simulink model "Task_No6_Thermal"  (R2023b)
settings: Solver=ode5  StartTime=0.0  StopTime=3600*24*7  FixedStep=1  RelTol=1e-3
InitFcn:
  | PARAMETERS;
StartFcn:
  | PARAMETERS;
values from neighbouring files (symbols this model uses):
  Conv_C_to_K = 273.15    [PARAMETERS.m]
  P_AC_AIR_FLOW = 1    [PARAMETERS.m]
  P_AREA_BATH = 2*4    (= 8)    [PARAMETERS.m]
  P_AREA_BDR1 = 3.87^2    (= 14.9769)    [PARAMETERS.m]
  P_AREA_BDR2 = 3.87*4.5    (= 17.415)    [PARAMETERS.m]
  P_AREA_EAST_WALL_BATH = 2*P_RM_HEIGHT - P_AREA_WIN_BATH    (= 3.7)    [PARAMETERS.m]
  P_AREA_EAST_WALL_BDR2 = 3.87*P_RM_HEIGHT - P_AREA_WIN_BDRS    (= 7.075)    [PARAMETERS.m]
  P_AREA_EAST_WALL_KIT = 4.13*P_RM_HEIGHT    (= 10.325)    [PARAMETERS.m]
  P_AREA_HALL = 2*6    (= 12)    [PARAMETERS.m]
  P_AREA_KIT = 4.13*4    (= 16.52)    [PARAMETERS.m]
  P_AREA_LVR = 4.13*6    (= 24.78)    [PARAMETERS.m]
  P_AREA_NORTH_WALL_BATH = 1.63*P_RM_HEIGHT    (= 4.075)    [PARAMETERS.m]
  P_AREA_NORTH_WALL_BDR1 = 3.87*P_RM_HEIGHT - P_AREA_WIN_BDRS    (= 7.075)    [PARAMETERS.m]
  P_AREA_NORTH_WALL_BDR2 = 4.5*P_RM_HEIGHT - P_AREA_WIN_BDRS    (= 8.65)    [PARAMETERS.m]
  P_AREA_OUTER_WALL_BATH = (1.63+2)*P_RM_HEIGHT - P_AREA_WIN_BATH    (= 7.775)    [PARAMETERS.m]
  P_AREA_OUTER_WALL_BDR1 = 3.87*2*P_RM_HEIGHT - P_AREA_WIN_BDRS    (= 16.75)    [PARAMETERS.m]
  P_AREA_OUTER_WALL_BDR2 = (4.5+3.87)*P_RM_HEIGHT - P_AREA_WIN_BDRS*2    (= 15.725)    [PARAMETERS.m]
  P_AREA_OUTER_WALL_HALL = 2*P_RM_HEIGHT - P_AREA_SING_DOOR    (= 2.9)    [PARAMETERS.m]
  P_AREA_OUTER_WALL_KIT = (4+4.13)*P_RM_HEIGHT - P_AREA_WIN_KIT    (= 13.725)    [PARAMETERS.m]
  P_AREA_OUTER_WALL_LVR = (4.13+6)*P_RM_HEIGHT - P_AREA_WIN_LVR    (= 14.325)    [PARAMETERS.m]
  P_AREA_SOUTH_WALL_KIT = 4*P_RM_HEIGHT - P_AREA_WIN_KIT    (= 3.4)    [PARAMETERS.m]
  P_AREA_SOUTH_WALL_LVR = 6*P_RM_HEIGHT - P_AREA_WIN_LVR    (= 4)    [PARAMETERS.m]
  P_AREA_WALL_BATH_KIT = 4*P_RM_HEIGHT    (= 10)    [PARAMETERS.m]
  P_AREA_WALL_BDR1_BDR2 = 3.87*P_RM_HEIGHT    (= 9.675)    [PARAMETERS.m]
  P_AREA_WALL_BDR1_HALL = 3.87*P_RM_HEIGHT - P_AREA_SING_DOOR    (= 7.575)    [PARAMETERS.m]
  P_AREA_WALL_BDR2_BATH = 2.37*P_RM_HEIGHT    (= 5.925)    [PARAMETERS.m]
  P_AREA_WALL_BDR2_HALL = 2.13*P_RM_HEIGHT - P_AREA_SING_DOOR    (= 3.225)    [PARAMETERS.m]
  P_AREA_WALL_HALL_BATH = 2*P_RM_HEIGHT - P_AREA_SING_DOOR    (= 2.9)    [PARAMETERS.m]
  P_AREA_WALL_HALL_LVR = 6*P_RM_HEIGHT - P_AREA_DBL_DOOR    (= 10.8)    [PARAMETERS.m]
  P_AREA_WALL_LVR_KIT = 4.13*P_RM_HEIGHT - P_AREA_DBL_DOOR    (= 6.125)    [PARAMETERS.m]
  P_AREA_WIN_BATH = P_H_WIN_NORM*P_W_WIN_BATH    (= 1.3)    [PARAMETERS.m]
  P_AREA_WIN_BDRS = P_H_WIN_NORM*P_W_WIN_BDRS    (= 2.6)    [PARAMETERS.m]
  P_AREA_WIN_KIT = P_H_WIN_DOOR*P_W_WIN_KIT    (= 6.6)    [PARAMETERS.m]
  P_AREA_WIN_LVR = P_H_WIN_DOOR*P_W_WIN_LVR    (= 11)    [PARAMETERS.m]
  P_CP_AIR = 1012    [PARAMETERS.m]
  P_DENSITY_BRICK = 2/(10^-3)    (= 2000)    [PARAMETERS.m]
  P_DENSITY_PUR = 150    [PARAMETERS.m]
  P_EM_GLASS = 0.94    [PARAMETERS.m]
  P_EM_WALL = 0.94    [PARAMETERS.m]
  P_HUMAN = 60    [PARAMETERS.m]
  P_M_WINDOW_SPEC = 20    [PARAMETERS.m]
  P_THICK_BRICK = 0.175    [PARAMETERS.m]
  P_THICK_PUR = P_THICK_WALL - P_THICK_BRICK    (= 0.125)    [PARAMETERS.m]
  T_COOLER = 12    [PARAMETERS.m]
  T_HEATER = 50    [PARAMETERS.m]
  T_INIT_BDR = 22    [PARAMETERS.m]
  T_INIT_OUT = 2.9    [PARAMETERS.m]
  U_CEIL = 1.1    [PARAMETERS.m]
  U_INNER_WALL_BR = 3    [PARAMETERS.m]
  U_INNER_WALL_PC = 0.6    [PARAMETERS.m]
  U_WALL = 0.32    [PARAMETERS.m]
  U_WINDOW = 3.0    (= 3)    [PARAMETERS.m]
undefined symbols (not defined in the file or in its folder): TBL_SOL_EAST_01, TBL_SOL_EAST_02, TBL_SOL_EAST_03, TBL_SOL_EAST_04, TBL_SOL_EAST_05, TBL_SOL_EAST_06, TBL_SOL_EAST_07, TBL_SOL_EAST_08, TBL_SOL_EAST_09, TBL_SOL_EAST_10, TBL_SOL_EAST_11, TBL_SOL_EAST_12, TBL_SOL_NORTH_01, TBL_SOL_NORTH_02, TBL_SOL_NORTH_03, TBL_SOL_NORTH_04, TBL_SOL_NORTH_05, TBL_SOL_NORTH_06, TBL_SOL_NORTH_07, TBL_SOL_NORTH_08, TBL_SOL_NORTH_09, TBL_SOL_NORTH_10, TBL_SOL_NORTH_11, TBL_SOL_NORTH_12, TBL_SOL_SOUTH_01, TBL_TEMP
libraries: fl_lib x135, nesl_utility x39, slpidlib x3
(part 2 of 3)

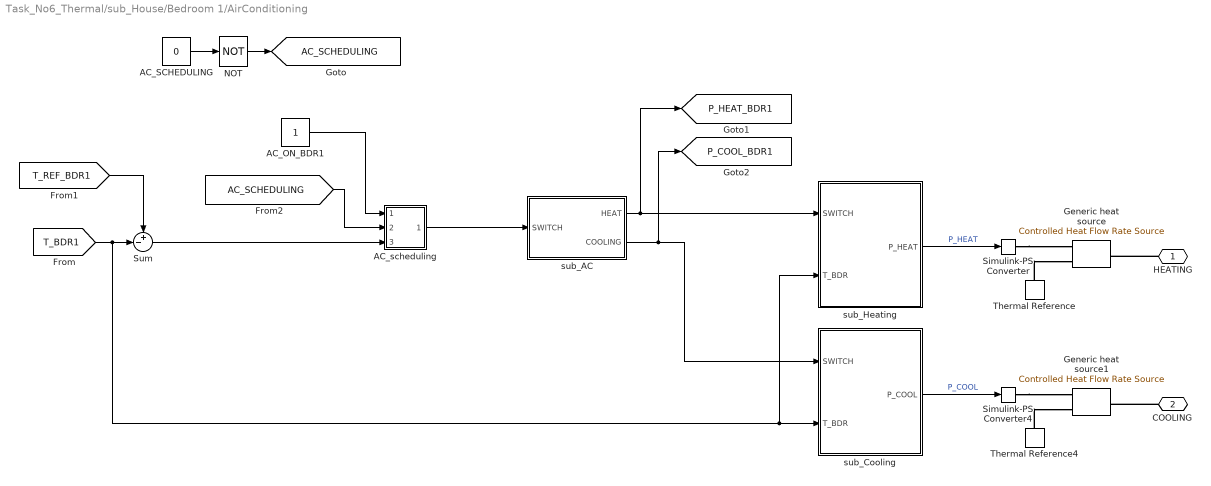
== system Task_No6_Thermal/sub_House/Bedroom 1/AirConditioning ==
  AC_ON_BDR1 : Constant
  AC_SCHEDULING : Constant  Value=0
  AC_scheduling : Subsystem
  Generic heat source : fl_lib/Thermal/Thermal Sources/Controlled Heat Flow Rate Source
  Generic heat source1 : fl_lib/Thermal/Thermal Sources/Controlled Heat Flow Rate Source
  NOT : Logic  Operator=NOT  IconShape=distinctive  AllPortsSameDT=off  OutDataTypeStr=boolean
  Simulink-PS Converter : nesl_utility/Simulink-PS Converter  PhysicalDomain=network_engine_domain  SubClassName=ps_input  LeftPortType=input  RightPortType=output  PseudoPeriodic=off  Frequencies=[]  NoiseDistribution=none  NoiseParameters=[]  Unit=1  AffineConversion=off  FilteringAndDerivatives=provide  SimscapeFilterOrder=1  InputFilterTimeConstant=0.001  UdotUserProvided=0
  Simulink-PS Converter4 : nesl_utility/Simulink-PS Converter  PhysicalDomain=network_engine_domain  SubClassName=ps_input  LeftPortType=input  RightPortType=output  PseudoPeriodic=off  Frequencies=[]  NoiseDistribution=none  NoiseParameters=[]  Unit=1  AffineConversion=off  FilteringAndDerivatives=provide  SimscapeFilterOrder=1  InputFilterTimeConstant=0.001  UdotUserProvided=0
  Sum : Sum  Inputs=+-|
  Thermal Reference : fl_lib/Thermal/Thermal Elements/Thermal Reference
  Thermal Reference4 : fl_lib/Thermal/Thermal Elements/Thermal Reference
  sub_AC : Subsystem
  sub_Cooling : Subsystem
  sub_Heating : Subsystem
  HEATING : PMIOPort  Side=Right
  COOLING : PMIOPort  Port=2  Side=Right
  tag scope: AC_SCHEDULING=global, P_COOL_BDR1=global, P_HEAT_BDR1=global
  wires:
  sub_AC/2(COOLING) -> [P_COOL_BDR1], sub_Cooling/1(SWITCH)
  sub_AC/1(HEAT) -> [P_HEAT_BDR1], sub_Heating/1(SWITCH)
  [T_BDR1] -> sub_Heating/2(T_BDR), sub_Cooling/2(T_BDR), Sum/2
  sub_Heating/1(P_HEAT) -> Simulink-PS Converter/1  "P_HEAT"
  sub_Cooling/1(P_COOL) -> Simulink-PS Converter4/1  "P_COOL"
  [T_REF_BDR1] -> Sum/1
  AC_ON_BDR1/1 -> AC_scheduling/1(In1)
  Sum/1 -> AC_scheduling/3(In2)
  AC_scheduling/1(Out1) -> sub_AC/1(SWITCH)
  AC_SCHEDULING/1 -> NOT/1
  [AC_SCHEDULING] -> AC_scheduling/2(In3)
  NOT/1 -> [AC_SCHEDULING]
  connections:
  Thermal Reference4/LConn1 -- Generic heat source1/RConn2
  Thermal Reference/LConn1 -- Generic heat source/RConn2
  Simulink-PS Converter4/RConn1 -- Generic heat source1/RConn1
  Simulink-PS Converter/RConn1 -- Generic heat source/RConn1
  HEATING/RConn1 -- Generic heat source/LConn1
  COOLING/RConn1 -- Generic heat source1/LConn1

== system Task_No6_Thermal/sub_House/Bedroom 1/Ceiling & Floor (BDR1<->Above & Below) ==
  Ceiling-InAir : fl_lib/Thermal/Thermal Elements/Thermal Resistance  resistance=1/(U_CEIL*P_AREA_BDR1) K/W  T_specify=off  T_priority=None  T=0 K  T_nominal_specify=off  T_nominal_unit=K  T_nominal_value=1  Q_specify=off  Q_priority=None  Q=0 W  Q_nominal_specify=off  Q_nominal_unit=W  Q_nominal_value=1
  Floor-InAir : fl_lib/Thermal/Thermal Elements/Thermal Resistance  resistance=1/(U_CEIL*P_AREA_BDR1) K/W  T_specify=off  T_priority=None  T=0 K  T_nominal_specify=off  T_nominal_unit=K  T_nominal_value=1  Q_specify=off  Q_priority=None  Q=0 W  Q_nominal_specify=off  Q_nominal_unit=W  Q_nominal_value=1
  Conn1 : PMIOPort  Side=Left
  Conn2 : PMIOPort  Port=2  Side=Right
  connections:
  Ceiling-InAir/RConn1 -- Conn2/RConn1 -- Floor-InAir/RConn1
  Ceiling-InAir/LConn1 -- Conn1/RConn1 -- Floor-InAir/LConn1

== system Task_No6_Thermal/sub_House/Bedroom 1/Heat source human ==
  Constant : Constant  Value=P_HUMAN
  Controlled Heat Flow Rate Source : fl_lib/Thermal/Thermal Sources/Controlled Heat Flow Rate Source
  Product : Product
  Simulink-PS Converter : nesl_utility/Simulink-PS Converter  PhysicalDomain=network_engine_domain  SubClassName=ps_input  LeftPortType=input  RightPortType=output  PseudoPeriodic=off  Frequencies=[]  NoiseDistribution=none  NoiseParameters=[]  Unit=1  AffineConversion=off  FilteringAndDerivatives=provide  SimscapeFilterOrder=1  InputFilterTimeConstant=0.001  UdotUserProvided=0
  Thermal Reference : fl_lib/Thermal/Thermal Elements/Thermal Reference
  Conn1 : PMIOPort  Side=Left
  wires:
  [N_BDR1] -> Product/1
  Constant/1 -> Product/2
  Product/1 -> Simulink-PS Converter/1
  connections:
  Thermal Reference/LConn1 -- Controlled Heat Flow Rate Source/RConn2
  Simulink-PS Converter/RConn1 -- Controlled Heat Flow Rate Source/RConn1
  Controlled Heat Flow Rate Source/LConn1 -- Conn1/RConn1

== system Task_No6_Thermal/sub_House/Bedroom 1/Inside Enivornment Temperature ==
  T_ENV : Inport
  Constant2 : Constant  Value=Conv_C_to_K
  Controlled Temperature Source : fl_lib/Thermal/Thermal Sources/Controlled Temperature Source
  Simulink-PS Converter1 : nesl_utility/Simulink-PS Converter  PhysicalDomain=network_engine_domain  SubClassName=ps_input  LeftPortType=input  RightPortType=output  PseudoPeriodic=off  Frequencies=[]  NoiseDistribution=none  NoiseParameters=[]  Unit=1  AffineConversion=off  FilteringAndDerivatives=provide  SimscapeFilterOrder=1  InputFilterTimeConstant=0.001  UdotUserProvided=0
  Sum : Sum  Inputs=|++
  Thermal Reference1 : fl_lib/Thermal/Thermal Elements/Thermal Reference
  Conn1 : PMIOPort  Side=Left
  wires:
  T_ENV/1 -> Sum/1
  Constant2/1 -> Sum/2
  Sum/1 -> Simulink-PS Converter1/1
  connections:
  Controlled Temperature Source/LConn1 -- Conn1/RConn1
  Simulink-PS Converter1/RConn1 -- Controlled Temperature Source/RConn1
  Thermal Reference1/LConn1 -- Controlled Temperature Source/RConn2

== system Task_No6_Thermal/sub_House/Bedroom 1/Outside Temperature ==
  T_OUT : Inport
  Constant2 : Constant  Value=Conv_C_to_K
  Controlled Temperature Source : fl_lib/Thermal/Thermal Sources/Controlled Temperature Source
  Simulink-PS Converter1 : nesl_utility/Simulink-PS Converter  PhysicalDomain=network_engine_domain  SubClassName=ps_input  LeftPortType=input  RightPortType=output  PseudoPeriodic=off  Frequencies=[]  NoiseDistribution=none  NoiseParameters=[]  Unit=1  AffineConversion=off  FilteringAndDerivatives=provide  SimscapeFilterOrder=1  InputFilterTimeConstant=0.001  UdotUserProvided=0
  Sum : Sum  Inputs=|++
  Thermal Reference1 : fl_lib/Thermal/Thermal Elements/Thermal Reference
  Conn1 : PMIOPort  Side=Left
  wires:
  Sum/1 -> Simulink-PS Converter1/1
  Constant2/1 -> Sum/2
  T_OUT/1 -> Sum/1
  connections:
  Thermal Reference1/LConn1 -- Controlled Temperature Source/RConn2
  Simulink-PS Converter1/RConn1 -- Controlled Temperature Source/RConn1
  Controlled Temperature Source/LConn1 -- Conn1/RConn1

== system Task_No6_Thermal/sub_House/Bedroom 1/SOLAR__WALL ==
  Constant : Constant  Value=P_AREA_NORTH_WALL_BDR1
  Constant1 : Constant  Value=P_EM_WALL
  Controlled Heat Flow Rate Source : fl_lib/Thermal/Thermal Sources/Controlled Heat Flow Rate Source
  Product : Product  Inputs=3
  Simulink-PS Converter : nesl_utility/Simulink-PS Converter  PhysicalDomain=network_engine_domain  SubClassName=ps_input  LeftPortType=input  RightPortType=output  PseudoPeriodic=off  Frequencies=[]  NoiseDistribution=none  NoiseParameters=[]  Unit=1  AffineConversion=off  FilteringAndDerivatives=provide  SimscapeFilterOrder=1  InputFilterTimeConstant=0.001  UdotUserProvided=0
  Thermal Reference : fl_lib/Thermal/Thermal Elements/Thermal Reference
  Conn1 : PMIOPort  Side=Left
  wires:
  Constant/1 -> Product/2
  Constant1/1 -> Product/1
  [SOL_NORTH] -> Product/3
  Product/1 -> Simulink-PS Converter/1
  connections:
  Controlled Heat Flow Rate Source/LConn1 -- Conn1/RConn1
  Simulink-PS Converter/RConn1 -- Controlled Heat Flow Rate Source/RConn1
  Thermal Reference/LConn1 -- Controlled Heat Flow Rate Source/RConn2

== system Task_No6_Thermal/sub_House/Bedroom 1/SOLAR__WINDOW ==
  Constant : Constant  Value=P_AREA_WIN_BDRS
  Constant1 : Constant  Value=P_EM_GLASS
  Controlled Heat Flow Rate Source : fl_lib/Thermal/Thermal Sources/Controlled Heat Flow Rate Source
  Product : Product  Inputs=3
  Simulink-PS Converter : nesl_utility/Simulink-PS Converter  PhysicalDomain=network_engine_domain  SubClassName=ps_input  LeftPortType=input  RightPortType=output  PseudoPeriodic=off  Frequencies=[]  NoiseDistribution=none  NoiseParameters=[]  Unit=1  AffineConversion=off  FilteringAndDerivatives=provide  SimscapeFilterOrder=1  InputFilterTimeConstant=0.001  UdotUserProvided=0
  Thermal Reference : fl_lib/Thermal/Thermal Elements/Thermal Reference
  Conn1 : PMIOPort  Side=Left
  wires:
  Product/1 -> Simulink-PS Converter/1
  [SOL_NORTH] -> Product/3
  Constant1/1 -> Product/1
  Constant/1 -> Product/2
  connections:
  Thermal Reference/LConn1 -- Controlled Heat Flow Rate Source/RConn2
  Simulink-PS Converter/RConn1 -- Controlled Heat Flow Rate Source/RConn1
  Controlled Heat Flow Rate Source/LConn1 -- Conn1/RConn1

== system Task_No6_Thermal/sub_House/Bedroom 1/TEMP_01 ==
  Constant2 : Constant  Value=Conv_C_to_K
  PS-Simulink Converter : nesl_utility/PS-Simulink Converter  PhysicalDomain=network_engine_domain  SubClassName=ps_output  LeftPortType=input  RightPortType=output  PseudoPeriodic=off  Frequencies=[]  VectorFormat=inherit  Unit=inherit  AffineConversion=off
  Sum : Sum  Inputs=|+-
  Temperature Sensor : fl_lib/Thermal/Thermal Sensors/Temperature Sensor  temperature_measure=foundation.enum.MeasurementReference.difference
  Thermal Reference2 : fl_lib/Thermal/Thermal Elements/Thermal Reference
  PS : PMIOPort  Side=Left
  Sim : Outport
  wires:
  Sum/1 -> Sim/1
  PS-Simulink Converter/1 -> Sum/1
  Constant2/1 -> Sum/2
  connections:
  Thermal Reference2/LConn1 -- Temperature Sensor/RConn1
  PS-Simulink Converter/LConn1 -- Temperature Sensor/RConn2
  PS/RConn1 -- Temperature Sensor/LConn1

== system Task_No6_Thermal/sub_House/Bedroom 1/Wall (BDR1<->Outside) ==
  InAir-Wall : fl_lib/Thermal/Thermal Elements/Thermal Resistance  resistance=1/(U_WALL*P_AREA_OUTER_WALL_BDR1)/2 K/W  T_specify=off  T_priority=None  T=0 K  T_nominal_specify=off  T_nominal_unit=K  T_nominal_value=1  Q_specify=off  Q_priority=None  Q=0 W  Q_nominal_specify=off  Q_nominal_unit=W  Q_nominal_value=1
  Thermal Mass of wall : fl_lib/Thermal/Thermal Elements/Thermal Mass  mass_type=foundation.enum.constant_variable.constant  mass=P_AREA_OUTER_WALL_BDR1*(P_THICK_BRICK*P_DENSITY_BRICK+P_THICK_PUR*P_DENSITY_PUR) kg  sp_heat=P_CP_WALL J/(K*kg)  mass_min=1e-6 kg  num_ports=foundation.enum.numPorts2.one  m_specify=off  m_priority=High  m=1 kg  m_nominal_specify=off  m_nominal_unit=kg  m_nominal_value=1  T_specify=on  T_priority=High  T=T_INIT_BDR degC  T_nominal_specify=off  T_nominal_unit=K  T_nominal_value=1  Q_specify=off  Q_priority=None  Q=0 W  Q_nominal_specify=off  Q_nominal_unit=W  Q_nominal_value=1
  Wall-OutAir : fl_lib/Thermal/Thermal Elements/Thermal Resistance  resistance=1/(U_WALL*P_AREA_OUTER_WALL_BDR1)/2 K/W  T_specify=off  T_priority=None  T=0 K  T_nominal_specify=off  T_nominal_unit=K  T_nominal_value=1  Q_specify=off  Q_priority=None  Q=0 W  Q_nominal_specify=off  Q_nominal_unit=W  Q_nominal_value=1
  Conn1 : PMIOPort  Side=Left
  Conn3 : PMIOPort  Port=2  Side=Right
  Conn2 : PMIOPort  Port=3  Side=Right
  connections:
  Conn1/RConn1 -- InAir-Wall/LConn1
  InAir-Wall/RConn1 -- Conn3/RConn1 -- Thermal Mass of wall/LConn1 -- Wall-OutAir/LConn1
  Wall-OutAir/RConn1 -- Conn2/RConn1

== system Task_No6_Thermal/sub_House/Bedroom 1/Window (BDR1<->Outside) ==
  InAir-Window : fl_lib/Thermal/Thermal Elements/Thermal Resistance  resistance=1/(U_WINDOW*P_AREA_WIN_BDRS)/2 K/W  T_specify=off  T_priority=None  T=0 K  T_nominal_specify=off  T_nominal_unit=K  T_nominal_value=1  Q_specify=off  Q_priority=None  Q=0 W  Q_nominal_specify=off  Q_nominal_unit=W  Q_nominal_value=1
  Thermal Mass of window : fl_lib/Thermal/Thermal Elements/Thermal Mass  mass_type=foundation.enum.constant_variable.constant  mass=P_M_WINDOW_SPEC*P_AREA_WIN_BDRS kg  sp_heat=P_CP_GLASS J/(K*kg)  mass_min=1e-6 kg  num_ports=foundation.enum.numPorts2.one  m_specify=off  m_priority=High  m=1 kg  m_nominal_specify=off  m_nominal_unit=kg  m_nominal_value=1  T_specify=on  T_priority=High  T=T_INIT_BDR degC  T_nominal_specify=off  T_nominal_unit=K  T_nominal_value=1  Q_specify=off  Q_priority=None  Q=0 W  Q_nominal_specify=off  Q_nominal_unit=W  Q_nominal_value=1
  Window-OutAir : fl_lib/Thermal/Thermal Elements/Thermal Resistance  resistance=1/(U_WINDOW*P_AREA_WIN_BDRS)/2 K/W  T_specify=off  T_priority=None  T=0 K  T_nominal_specify=off  T_nominal_unit=K  T_nominal_value=1  Q_specify=off  Q_priority=None  Q=0 W  Q_nominal_specify=off  Q_nominal_unit=W  Q_nominal_value=1
  Conn1 : PMIOPort  Side=Right
  Conn2 : PMIOPort  Port=2  Side=Left
  Conn3 : PMIOPort  Port=3  Side=Right
  connections:
  Window-OutAir/LConn1 -- Thermal Mass of window/LConn1 -- Conn3/RConn1 -- InAir-Window/RConn1
  Conn1/RConn1 -- Window-OutAir/RConn1
  Conn2/RConn1 -- InAir-Window/LConn1

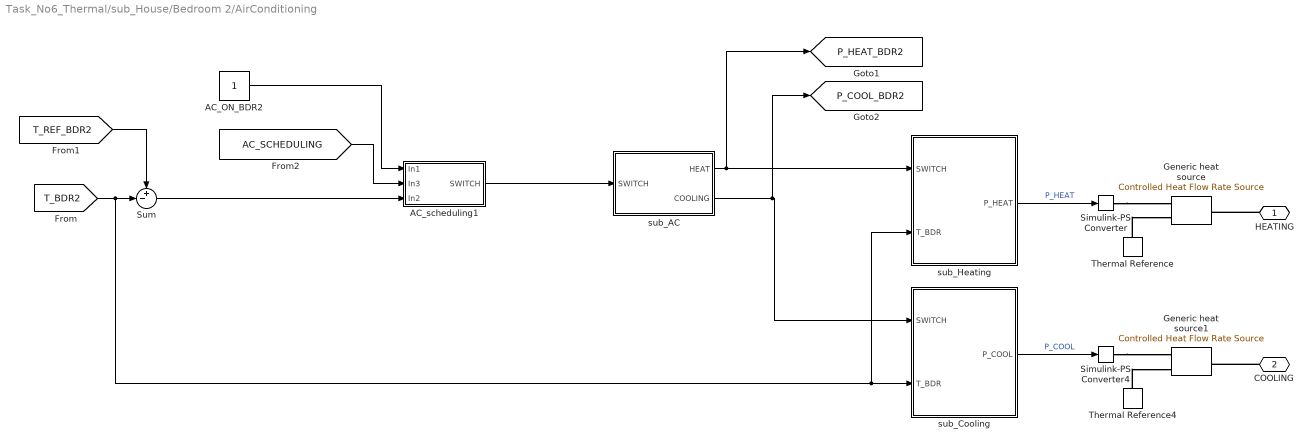
== system Task_No6_Thermal/sub_House/Bedroom 2/AirConditioning ==
  AC_ON_BDR2 : Constant
  AC_scheduling1 : Subsystem
  Generic heat source : fl_lib/Thermal/Thermal Sources/Controlled Heat Flow Rate Source
  Generic heat source1 : fl_lib/Thermal/Thermal Sources/Controlled Heat Flow Rate Source
  Simulink-PS Converter : nesl_utility/Simulink-PS Converter  PhysicalDomain=network_engine_domain  SubClassName=ps_input  LeftPortType=input  RightPortType=output  PseudoPeriodic=off  Frequencies=[]  NoiseDistribution=none  NoiseParameters=[]  Unit=1  AffineConversion=off  FilteringAndDerivatives=provide  SimscapeFilterOrder=1  InputFilterTimeConstant=0.001  UdotUserProvided=0
  Simulink-PS Converter4 : nesl_utility/Simulink-PS Converter  PhysicalDomain=network_engine_domain  SubClassName=ps_input  LeftPortType=input  RightPortType=output  PseudoPeriodic=off  Frequencies=[]  NoiseDistribution=none  NoiseParameters=[]  Unit=1  AffineConversion=off  FilteringAndDerivatives=provide  SimscapeFilterOrder=1  InputFilterTimeConstant=0.001  UdotUserProvided=0
  Sum : Sum  Inputs=+-|
  Thermal Reference : fl_lib/Thermal/Thermal Elements/Thermal Reference
  Thermal Reference4 : fl_lib/Thermal/Thermal Elements/Thermal Reference
  sub_AC : Subsystem
  sub_Cooling : Subsystem
  sub_Heating : Subsystem
  HEATING : PMIOPort  Side=Right
  COOLING : PMIOPort  Port=2  Side=Right
  tag scope: P_COOL_BDR2=global, P_HEAT_BDR2=global
  wires:
  sub_AC/2(COOLING) -> [P_COOL_BDR2], sub_Cooling/1(SWITCH)
  sub_AC/1(HEAT) -> [P_HEAT_BDR2], sub_Heating/1(SWITCH)
  [T_BDR2] -> sub_Heating/2(T_BDR), sub_Cooling/2(T_BDR), Sum/2
  sub_Heating/1(P_HEAT) -> Simulink-PS Converter/1  "P_HEAT"
  sub_Cooling/1(P_COOL) -> Simulink-PS Converter4/1  "P_COOL"
  [T_REF_BDR2] -> Sum/1
  Sum/1 -> AC_scheduling1/3(In2)
  AC_scheduling1/1(SWITCH) -> sub_AC/1(SWITCH)
  AC_ON_BDR2/1 -> AC_scheduling1/1(In1)
  [AC_SCHEDULING] -> AC_scheduling1/2(In3)
  connections:
  Thermal Reference4/LConn1 -- Generic heat source1/RConn2
  Thermal Reference/LConn1 -- Generic heat source/RConn2
  Simulink-PS Converter4/RConn1 -- Generic heat source1/RConn1
  Simulink-PS Converter/RConn1 -- Generic heat source/RConn1
  HEATING/RConn1 -- Generic heat source/LConn1
  COOLING/RConn1 -- Generic heat source1/LConn1

== system Task_No6_Thermal/sub_House/Bedroom 2/Ceiling & Floor (BDR2<->Above & Below) ==
  Ceiling-InAir : fl_lib/Thermal/Thermal Elements/Thermal Resistance  resistance=1/(U_CEIL*P_AREA_BDR2) K/W  T_specify=off  T_priority=None  T=0 K  T_nominal_specify=off  T_nominal_unit=K  T_nominal_value=1  Q_specify=off  Q_priority=None  Q=0 W  Q_nominal_specify=off  Q_nominal_unit=W  Q_nominal_value=1
  Floor-InAir : fl_lib/Thermal/Thermal Elements/Thermal Resistance  resistance=1/(U_CEIL*P_AREA_BDR2) K/W  T_specify=off  T_priority=None  T=0 K  T_nominal_specify=off  T_nominal_unit=K  T_nominal_value=1  Q_specify=off  Q_priority=None  Q=0 W  Q_nominal_specify=off  Q_nominal_unit=W  Q_nominal_value=1
  Conn1 : PMIOPort  Side=Left
  Conn2 : PMIOPort  Port=2  Side=Right
  connections:
  Conn1/RConn1 -- Ceiling-InAir/LConn1 -- Floor-InAir/LConn1
  Conn2/RConn1 -- Ceiling-InAir/RConn1 -- Floor-InAir/RConn1

== system Task_No6_Thermal/sub_House/Bedroom 2/Heat source human ==
  Constant : Constant  Value=P_HUMAN
  Controlled Heat Flow Rate Source : fl_lib/Thermal/Thermal Sources/Controlled Heat Flow Rate Source
  Product : Product
  Simulink-PS Converter : nesl_utility/Simulink-PS Converter  PhysicalDomain=network_engine_domain  SubClassName=ps_input  LeftPortType=input  RightPortType=output  PseudoPeriodic=off  Frequencies=[]  NoiseDistribution=none  NoiseParameters=[]  Unit=1  AffineConversion=off  FilteringAndDerivatives=provide  SimscapeFilterOrder=1  InputFilterTimeConstant=0.001  UdotUserProvided=0
  Thermal Reference : fl_lib/Thermal/Thermal Elements/Thermal Reference
  Conn1 : PMIOPort  Side=Left
  wires:
  [N_BDR2] -> Product/1
  Constant/1 -> Product/2
  Product/1 -> Simulink-PS Converter/1
  connections:
  Thermal Reference/LConn1 -- Controlled Heat Flow Rate Source/RConn2
  Simulink-PS Converter/RConn1 -- Controlled Heat Flow Rate Source/RConn1
  Controlled Heat Flow Rate Source/LConn1 -- Conn1/RConn1

== system Task_No6_Thermal/sub_House/Bedroom 2/Inside Enivornment Temperature ==
  T_ENV : Inport
  Constant2 : Constant  Value=Conv_C_to_K
  Controlled Temperature Source : fl_lib/Thermal/Thermal Sources/Controlled Temperature Source
  Simulink-PS Converter1 : nesl_utility/Simulink-PS Converter  PhysicalDomain=network_engine_domain  SubClassName=ps_input  LeftPortType=input  RightPortType=output  PseudoPeriodic=off  Frequencies=[]  NoiseDistribution=none  NoiseParameters=[]  Unit=1  AffineConversion=off  FilteringAndDerivatives=provide  SimscapeFilterOrder=1  InputFilterTimeConstant=0.001  UdotUserProvided=0
  Sum : Sum  Inputs=|++
  Thermal Reference1 : fl_lib/Thermal/Thermal Elements/Thermal Reference
  Conn1 : PMIOPort  Side=Left
  wires:
  T_ENV/1 -> Sum/1
  Constant2/1 -> Sum/2
  Sum/1 -> Simulink-PS Converter1/1
  connections:
  Controlled Temperature Source/LConn1 -- Conn1/RConn1
  Simulink-PS Converter1/RConn1 -- Controlled Temperature Source/RConn1
  Thermal Reference1/LConn1 -- Controlled Temperature Source/RConn2

== system Task_No6_Thermal/sub_House/Bedroom 2/Outside Temperature ==
  T_OUT : Inport
  Constant2 : Constant  Value=Conv_C_to_K
  Controlled Temperature Source : fl_lib/Thermal/Thermal Sources/Controlled Temperature Source
  Simulink-PS Converter1 : nesl_utility/Simulink-PS Converter  PhysicalDomain=network_engine_domain  SubClassName=ps_input  LeftPortType=input  RightPortType=output  PseudoPeriodic=off  Frequencies=[]  NoiseDistribution=none  NoiseParameters=[]  Unit=1  AffineConversion=off  FilteringAndDerivatives=provide  SimscapeFilterOrder=1  InputFilterTimeConstant=0.001  UdotUserProvided=0
  Sum : Sum  Inputs=|++
  Thermal Reference1 : fl_lib/Thermal/Thermal Elements/Thermal Reference
  Conn1 : PMIOPort  Side=Left
  wires:
  Sum/1 -> Simulink-PS Converter1/1
  Constant2/1 -> Sum/2
  T_OUT/1 -> Sum/1
  connections:
  Thermal Reference1/LConn1 -- Controlled Temperature Source/RConn2
  Simulink-PS Converter1/RConn1 -- Controlled Temperature Source/RConn1
  Controlled Temperature Source/LConn1 -- Conn1/RConn1

== system Task_No6_Thermal/sub_House/Bedroom 2/SOLAR__WALL ==
  Add : Sum
  Constant : Constant  Value=P_AREA_NORTH_WALL_BDR2
  Constant1 : Constant  Value=P_EM_WALL
  Constant2 : Constant  Value=P_AREA_EAST_WALL_BDR2
  Constant3 : Constant  Value=P_EM_WALL
  Controlled Heat Flow Rate Source : fl_lib/Thermal/Thermal Sources/Controlled Heat Flow Rate Source
  Product : Product  Inputs=3
  Product1 : Product  Inputs=3
  Simulink-PS Converter : nesl_utility/Simulink-PS Converter  PhysicalDomain=network_engine_domain  SubClassName=ps_input  LeftPortType=input  RightPortType=output  PseudoPeriodic=off  Frequencies=[]  NoiseDistribution=none  NoiseParameters=[]  Unit=1  AffineConversion=off  FilteringAndDerivatives=provide  SimscapeFilterOrder=1  InputFilterTimeConstant=0.001  UdotUserProvided=0
  Thermal Reference : fl_lib/Thermal/Thermal Elements/Thermal Reference
  Conn1 : PMIOPort  Side=Left
  wires:
  Constant/1 -> Product/2
  Constant1/1 -> Product/1
  [SOL_NORTH] -> Product/3
  Product/1 -> Add/1
  Constant3/1 -> Product1/1
  [SOL_EAST] -> Product1/3
  Constant2/1 -> Product1/2
  Add/1 -> Simulink-PS Converter/1
  Product1/1 -> Add/2
  connections:
  Controlled Heat Flow Rate Source/LConn1 -- Conn1/RConn1
  Simulink-PS Converter/RConn1 -- Controlled Heat Flow Rate Source/RConn1
  Thermal Reference/LConn1 -- Controlled Heat Flow Rate Source/RConn2

== system Task_No6_Thermal/sub_House/Bedroom 2/SOLAR__WINDOW ==
  Add : Sum
  Constant : Constant  Value=P_AREA_WIN_BDRS
  Constant1 : Constant  Value=P_EM_GLASS
  Constant2 : Constant  Value=P_AREA_WIN_BDRS
  Constant3 : Constant  Value=P_EM_GLASS
  Controlled Heat Flow Rate Source : fl_lib/Thermal/Thermal Sources/Controlled Heat Flow Rate Source
  Product : Product  Inputs=3
  Product1 : Product  Inputs=3
  Simulink-PS Converter : nesl_utility/Simulink-PS Converter  PhysicalDomain=network_engine_domain  SubClassName=ps_input  LeftPortType=input  RightPortType=output  PseudoPeriodic=off  Frequencies=[]  NoiseDistribution=none  NoiseParameters=[]  Unit=1  AffineConversion=off  FilteringAndDerivatives=provide  SimscapeFilterOrder=1  InputFilterTimeConstant=0.001  UdotUserProvided=0
  Thermal Reference : fl_lib/Thermal/Thermal Elements/Thermal Reference
  Conn1 : PMIOPort  Side=Left
  wires:
  Product/1 -> Add/1
  [SOL_NORTH] -> Product/3
  Constant1/1 -> Product/1
  Constant/1 -> Product/2
  Constant2/1 -> Product1/2
  Constant3/1 -> Product1/1
  [SOL_EAST] -> Product1/3
  Add/1 -> Simulink-PS Converter/1
  Product1/1 -> Add/2
  connections:
  Thermal Reference/LConn1 -- Controlled Heat Flow Rate Source/RConn2
  Simulink-PS Converter/RConn1 -- Controlled Heat Flow Rate Source/RConn1
  Controlled Heat Flow Rate Source/LConn1 -- Conn1/RConn1

== system Task_No6_Thermal/sub_House/Bedroom 2/TEMP_01 ==
  Constant2 : Constant  Value=Conv_C_to_K
  PS-Simulink Converter : nesl_utility/PS-Simulink Converter  PhysicalDomain=network_engine_domain  SubClassName=ps_output  LeftPortType=input  RightPortType=output  PseudoPeriodic=off  Frequencies=[]  VectorFormat=inherit  Unit=inherit  AffineConversion=off
  Sum : Sum  Inputs=|+-
  Temperature Sensor : fl_lib/Thermal/Thermal Sensors/Temperature Sensor  temperature_measure=foundation.enum.MeasurementReference.difference
  Thermal Reference2 : fl_lib/Thermal/Thermal Elements/Thermal Reference
  PS : PMIOPort  Side=Left
  Sim : Outport
  wires:
  Constant2/1 -> Sum/2
  PS-Simulink Converter/1 -> Sum/1
  Sum/1 -> Sim/1
  connections:
  PS/RConn1 -- Temperature Sensor/LConn1
  PS-Simulink Converter/LConn1 -- Temperature Sensor/RConn2
  Thermal Reference2/LConn1 -- Temperature Sensor/RConn1

== system Task_No6_Thermal/sub_House/Bedroom 2/Wall (BDR2<->Outside) ==
  InAir-Wall : fl_lib/Thermal/Thermal Elements/Thermal Resistance  resistance=1/(U_WALL*P_AREA_OUTER_WALL_BDR2)/2 K/W  T_specify=off  T_priority=None  T=0 K  T_nominal_specify=off  T_nominal_unit=K  T_nominal_value=1  Q_specify=off  Q_priority=None  Q=0 W  Q_nominal_specify=off  Q_nominal_unit=W  Q_nominal_value=1
  Thermal Mass of wall : fl_lib/Thermal/Thermal Elements/Thermal Mass  mass_type=foundation.enum.constant_variable.constant  mass=P_AREA_OUTER_WALL_BDR2*(P_THICK_BRICK*P_DENSITY_BRICK+P_THICK_PUR*P_DENSITY_PUR) kg  sp_heat=P_CP_WALL J/(K*kg)  mass_min=1e-6 kg  num_ports=foundation.enum.numPorts2.one  m_specify=off  m_priority=High  m=1 kg  m_nominal_specify=off  m_nominal_unit=kg  m_nominal_value=1  T_specify=on  T_priority=High  T=T_INIT_BDR degC  T_nominal_specify=off  T_nominal_unit=K  T_nominal_value=1  Q_specify=off  Q_priority=None  Q=0 W  Q_nominal_specify=off  Q_nominal_unit=W  Q_nominal_value=1
  Wall-OutAir : fl_lib/Thermal/Thermal Elements/Thermal Resistance  resistance=1/(U_WALL*P_AREA_OUTER_WALL_BDR2)/2 K/W  T_specify=off  T_priority=None  T=0 K  T_nominal_specify=off  T_nominal_unit=K  T_nominal_value=1  Q_specify=off  Q_priority=None  Q=0 W  Q_nominal_specify=off  Q_nominal_unit=W  Q_nominal_value=1
  Conn1 : PMIOPort  Side=Left
  Conn3 : PMIOPort  Port=2  Side=Right
  Conn2 : PMIOPort  Port=3  Side=Right
  connections:
  Wall-OutAir/RConn1 -- Conn2/RConn1
  Wall-OutAir/LConn1 -- Conn3/RConn1 -- Thermal Mass of wall/LConn1 -- InAir-Wall/RConn1
  Conn1/RConn1 -- InAir-Wall/LConn1

== system Task_No6_Thermal/sub_House/Bedroom 2/Window (BDR2<->Outside) ==
  InAir-Window : fl_lib/Thermal/Thermal Elements/Thermal Resistance  resistance=1/(U_WINDOW*P_AREA_WIN_BDRS*2)/2 K/W  T_specify=off  T_priority=None  T=0 K  T_nominal_specify=off  T_nominal_unit=K  T_nominal_value=1  Q_specify=off  Q_priority=None  Q=0 W  Q_nominal_specify=off  Q_nominal_unit=W  Q_nominal_value=1
  Thermal Mass of window : fl_lib/Thermal/Thermal Elements/Thermal Mass  mass_type=foundation.enum.constant_variable.constant  mass=P_M_WINDOW_SPEC*P_AREA_WIN_BDRS*2 kg  sp_heat=P_CP_GLASS J/(K*kg)  mass_min=1e-6 kg  num_ports=foundation.enum.numPorts2.one  m_specify=off  m_priority=High  m=1 kg  m_nominal_specify=off  m_nominal_unit=kg  m_nominal_value=1  T_specify=on  T_priority=High  T=T_INIT_BDR degC  T_nominal_specify=off  T_nominal_unit=K  T_nominal_value=1  Q_specify=off  Q_priority=None  Q=0 W  Q_nominal_specify=off  Q_nominal_unit=W  Q_nominal_value=1
  Window-OutAir : fl_lib/Thermal/Thermal Elements/Thermal Resistance  resistance=1/(U_WINDOW*P_AREA_WIN_BDRS*2)/2 K/W  T_specify=off  T_priority=None  T=0 K  T_nominal_specify=off  T_nominal_unit=K  T_nominal_value=1  Q_specify=off  Q_priority=None  Q=0 W  Q_nominal_specify=off  Q_nominal_unit=W  Q_nominal_value=1
  Conn1 : PMIOPort  Side=Right
  Conn2 : PMIOPort  Port=2  Side=Left
  Conn3 : PMIOPort  Port=3  Side=Right
  connections:
  Conn2/RConn1 -- InAir-Window/LConn1
  Conn1/RConn1 -- Window-OutAir/RConn1
  InAir-Window/RConn1 -- Thermal Mass of window/LConn1 -- Conn3/RConn1 -- Window-OutAir/LConn1

== system Task_No6_Thermal/sub_House/Hallway/Ceiling & Floor (Hall<->Above & Below) ==
  Ceiling-InAir : fl_lib/Thermal/Thermal Elements/Thermal Resistance  resistance=1/(U_CEIL*P_AREA_HALL) K/W  T_specify=off  T_priority=None  T=0 K  T_nominal_specify=off  T_nominal_unit=K  T_nominal_value=1  Q_specify=off  Q_priority=None  Q=0 W  Q_nominal_specify=off  Q_nominal_unit=W  Q_nominal_value=1
  Floor-InAir : fl_lib/Thermal/Thermal Elements/Thermal Resistance  resistance=1/(U_CEIL*P_AREA_HALL) K/W  T_specify=off  T_priority=None  T=0 K  T_nominal_specify=off  T_nominal_unit=K  T_nominal_value=1  Q_specify=off  Q_priority=None  Q=0 W  Q_nominal_specify=off  Q_nominal_unit=W  Q_nominal_value=1
  Conn1 : PMIOPort  Side=Left
  Conn2 : PMIOPort  Port=2  Side=Right
  connections:
  Floor-InAir/RConn1 -- Ceiling-InAir/RConn1 -- Conn2/RConn1
  Floor-InAir/LConn1 -- Ceiling-InAir/LConn1 -- Conn1/RConn1

== system Task_No6_Thermal/sub_House/Hallway/Inside Enivornment Temperature ==
  T_ENV : Inport
  Constant2 : Constant  Value=Conv_C_to_K
  Controlled Temperature Source : fl_lib/Thermal/Thermal Sources/Controlled Temperature Source
  Simulink-PS Converter1 : nesl_utility/Simulink-PS Converter  PhysicalDomain=network_engine_domain  SubClassName=ps_input  LeftPortType=input  RightPortType=output  PseudoPeriodic=off  Frequencies=[]  NoiseDistribution=none  NoiseParameters=[]  Unit=1  AffineConversion=off  FilteringAndDerivatives=provide  SimscapeFilterOrder=1  InputFilterTimeConstant=0.001  UdotUserProvided=0
  Sum : Sum  Inputs=|++
  Thermal Reference1 : fl_lib/Thermal/Thermal Elements/Thermal Reference
  Conn1 : PMIOPort  Side=Left
  wires:
  T_ENV/1 -> Sum/1
  Constant2/1 -> Sum/2
  Sum/1 -> Simulink-PS Converter1/1
  connections:
  Controlled Temperature Source/LConn1 -- Conn1/RConn1
  Simulink-PS Converter1/RConn1 -- Controlled Temperature Source/RConn1
  Thermal Reference1/LConn1 -- Controlled Temperature Source/RConn2

== system Task_No6_Thermal/sub_House/Hallway/Outside Temperature ==
  T_OUT : Inport
  Constant2 : Constant  Value=Conv_C_to_K
  Controlled Temperature Source : fl_lib/Thermal/Thermal Sources/Controlled Temperature Source
  Simulink-PS Converter1 : nesl_utility/Simulink-PS Converter  PhysicalDomain=network_engine_domain  SubClassName=ps_input  LeftPortType=input  RightPortType=output  PseudoPeriodic=off  Frequencies=[]  NoiseDistribution=none  NoiseParameters=[]  Unit=1  AffineConversion=off  FilteringAndDerivatives=provide  SimscapeFilterOrder=1  InputFilterTimeConstant=0.001  UdotUserProvided=0
  Sum : Sum  Inputs=|++
  Thermal Reference1 : fl_lib/Thermal/Thermal Elements/Thermal Reference
  Conn1 : PMIOPort  Side=Left
  wires:
  Sum/1 -> Simulink-PS Converter1/1
  Constant2/1 -> Sum/2
  T_OUT/1 -> Sum/1
  connections:
  Thermal Reference1/LConn1 -- Controlled Temperature Source/RConn2
  Simulink-PS Converter1/RConn1 -- Controlled Temperature Source/RConn1
  Controlled Temperature Source/LConn1 -- Conn1/RConn1

== system Task_No6_Thermal/sub_House/Hallway/TEMP_01 ==
  Constant2 : Constant  Value=Conv_C_to_K
  PS-Simulink Converter : nesl_utility/PS-Simulink Converter  PhysicalDomain=network_engine_domain  SubClassName=ps_output  LeftPortType=input  RightPortType=output  PseudoPeriodic=off  Frequencies=[]  VectorFormat=inherit  Unit=inherit  AffineConversion=off
  Sum : Sum  Inputs=|+-
  Temperature Sensor : fl_lib/Thermal/Thermal Sensors/Temperature Sensor  temperature_measure=foundation.enum.MeasurementReference.difference
  Thermal Reference2 : fl_lib/Thermal/Thermal Elements/Thermal Reference
  PS : PMIOPort  Side=Left
  Sim : Outport
  wires:
  Sum/1 -> Sim/1
  PS-Simulink Converter/1 -> Sum/1
  Constant2/1 -> Sum/2
  connections:
  Thermal Reference2/LConn1 -- Temperature Sensor/RConn1
  PS-Simulink Converter/LConn1 -- Temperature Sensor/RConn2
  PS/RConn1 -- Temperature Sensor/LConn1

== system Task_No6_Thermal/sub_House/Hallway/Wall (Hall<->Outside) ==
  InAir-Wall : fl_lib/Thermal/Thermal Elements/Thermal Resistance  resistance=1/(U_WALL*P_AREA_OUTER_WALL_HALL)/2 K/W  T_specify=off  T_priority=None  T=0 K  T_nominal_specify=off  T_nominal_unit=K  T_nominal_value=1  Q_specify=off  Q_priority=None  Q=0 W  Q_nominal_specify=off  Q_nominal_unit=W  Q_nominal_value=1
  Thermal Mass of wall : fl_lib/Thermal/Thermal Elements/Thermal Mass  mass_type=foundation.enum.constant_variable.constant  mass=P_AREA_OUTER_WALL_HALL*(P_THICK_BRICK*P_DENSITY_BRICK+P_THICK_PUR*P_DENSITY_PUR) kg  sp_heat=P_CP_WALL J/(K*kg)  mass_min=1e-6 kg  num_ports=foundation.enum.numPorts2.one  m_specify=off  m_priority=High  m=1 kg  m_nominal_specify=off  m_nominal_unit=kg  m_nominal_value=1  T_specify=on  T_priority=High  T=T_INIT_BDR degC  T_nominal_specify=off  T_nominal_unit=K  T_nominal_value=1  Q_specify=off  Q_priority=None  Q=0 W  Q_nominal_specify=off  Q_nominal_unit=W  Q_nominal_value=1
  Wall-OutAir : fl_lib/Thermal/Thermal Elements/Thermal Resistance  resistance=1/(U_WALL*P_AREA_OUTER_WALL_HALL)/2 K/W  T_specify=off  T_priority=None  T=0 K  T_nominal_specify=off  T_nominal_unit=K  T_nominal_value=1  Q_specify=off  Q_priority=None  Q=0 W  Q_nominal_specify=off  Q_nominal_unit=W  Q_nominal_value=1
  Conn1 : PMIOPort  Side=Left
  Conn2 : PMIOPort  Port=2  Side=Right
  connections:
  Conn1/RConn1 -- InAir-Wall/LConn1
  InAir-Wall/RConn1 -- Thermal Mass of wall/LConn1 -- Wall-OutAir/LConn1
  Wall-OutAir/RConn1 -- Conn2/RConn1

== system Task_No6_Thermal/sub_House/Kitchen/Ceiling & Floor (KIT<->Above & Below) ==
  Ceiling-InAir : fl_lib/Thermal/Thermal Elements/Thermal Resistance  resistance=1/(U_CEIL*P_AREA_KIT) K/W  T_specify=off  T_priority=None  T=0 K  T_nominal_specify=off  T_nominal_unit=K  T_nominal_value=1  Q_specify=off  Q_priority=None  Q=0 W  Q_nominal_specify=off  Q_nominal_unit=W  Q_nominal_value=1
  Floor-InAir : fl_lib/Thermal/Thermal Elements/Thermal Resistance  resistance=1/(U_CEIL*P_AREA_KIT) K/W  T_specify=off  T_priority=None  T=0 K  T_nominal_specify=off  T_nominal_unit=K  T_nominal_value=1  Q_specify=off  Q_priority=None  Q=0 W  Q_nominal_specify=off  Q_nominal_unit=W  Q_nominal_value=1
  Conn1 : PMIOPort  Side=Left
  Conn2 : PMIOPort  Port=2  Side=Right
  connections:
  Floor-InAir/RConn1 -- Ceiling-InAir/RConn1 -- Conn2/RConn1
  Floor-InAir/LConn1 -- Ceiling-InAir/LConn1 -- Conn1/RConn1

== system Task_No6_Thermal/sub_House/Kitchen/Heat source human ==
  Constant : Constant  Value=P_HUMAN
  Controlled Heat Flow Rate Source : fl_lib/Thermal/Thermal Sources/Controlled Heat Flow Rate Source
  Product : Product
  Simulink-PS Converter : nesl_utility/Simulink-PS Converter  PhysicalDomain=network_engine_domain  SubClassName=ps_input  LeftPortType=input  RightPortType=output  PseudoPeriodic=off  Frequencies=[]  NoiseDistribution=none  NoiseParameters=[]  Unit=1  AffineConversion=off  FilteringAndDerivatives=provide  SimscapeFilterOrder=1  InputFilterTimeConstant=0.001  UdotUserProvided=0
  Thermal Reference : fl_lib/Thermal/Thermal Elements/Thermal Reference
  Conn1 : PMIOPort  Side=Left
  wires:
  [N_KIT] -> Product/1
  Constant/1 -> Product/2
  Product/1 -> Simulink-PS Converter/1
  connections:
  Thermal Reference/LConn1 -- Controlled Heat Flow Rate Source/RConn2
  Simulink-PS Converter/RConn1 -- Controlled Heat Flow Rate Source/RConn1
  Controlled Heat Flow Rate Source/LConn1 -- Conn1/RConn1

== system Task_No6_Thermal/sub_House/Kitchen/Inside Enivornment Temperature ==
  T_ENV : Inport
  Constant2 : Constant  Value=Conv_C_to_K
  Controlled Temperature Source : fl_lib/Thermal/Thermal Sources/Controlled Temperature Source
  Simulink-PS Converter1 : nesl_utility/Simulink-PS Converter  PhysicalDomain=network_engine_domain  SubClassName=ps_input  LeftPortType=input  RightPortType=output  PseudoPeriodic=off  Frequencies=[]  NoiseDistribution=none  NoiseParameters=[]  Unit=1  AffineConversion=off  FilteringAndDerivatives=provide  SimscapeFilterOrder=1  InputFilterTimeConstant=0.001  UdotUserProvided=0
  Sum : Sum  Inputs=|++
  Thermal Reference1 : fl_lib/Thermal/Thermal Elements/Thermal Reference
  Conn1 : PMIOPort  Side=Left
  wires:
  T_ENV/1 -> Sum/1
  Constant2/1 -> Sum/2
  Sum/1 -> Simulink-PS Converter1/1
  connections:
  Controlled Temperature Source/LConn1 -- Conn1/RConn1
  Simulink-PS Converter1/RConn1 -- Controlled Temperature Source/RConn1
  Thermal Reference1/LConn1 -- Controlled Temperature Source/RConn2

== system Task_No6_Thermal/sub_House/Kitchen/Outside Temperature ==
  T_OUT : Inport
  Constant2 : Constant  Value=Conv_C_to_K
  Controlled Temperature Source : fl_lib/Thermal/Thermal Sources/Controlled Temperature Source
  Simulink-PS Converter1 : nesl_utility/Simulink-PS Converter  PhysicalDomain=network_engine_domain  SubClassName=ps_input  LeftPortType=input  RightPortType=output  PseudoPeriodic=off  Frequencies=[]  NoiseDistribution=none  NoiseParameters=[]  Unit=1  AffineConversion=off  FilteringAndDerivatives=provide  SimscapeFilterOrder=1  InputFilterTimeConstant=0.001  UdotUserProvided=0
  Sum : Sum  Inputs=|++
  Thermal Reference1 : fl_lib/Thermal/Thermal Elements/Thermal Reference
  Conn1 : PMIOPort  Side=Left
  wires:
  Sum/1 -> Simulink-PS Converter1/1
  Constant2/1 -> Sum/2
  T_OUT/1 -> Sum/1
  connections:
  Thermal Reference1/LConn1 -- Controlled Temperature Source/RConn2
  Simulink-PS Converter1/RConn1 -- Controlled Temperature Source/RConn1
  Controlled Temperature Source/LConn1 -- Conn1/RConn1

== system Task_No6_Thermal/sub_House/Kitchen/SOLAR__WALL ==
  Add : Sum
  Constant : Constant  Value=P_AREA_EAST_WALL_KIT
  Constant1 : Constant  Value=P_EM_WALL
  Constant2 : Constant  Value=P_AREA_SOUTH_WALL_KIT
  Constant3 : Constant  Value=P_EM_WALL
  Controlled Heat Flow Rate Source : fl_lib/Thermal/Thermal Sources/Controlled Heat Flow Rate Source
  Product : Product  Inputs=3
  Product1 : Product  Inputs=3
  Simulink-PS Converter : nesl_utility/Simulink-PS Converter  PhysicalDomain=network_engine_domain  SubClassName=ps_input  LeftPortType=input  RightPortType=output  PseudoPeriodic=off  Frequencies=[]  NoiseDistribution=none  NoiseParameters=[]  Unit=1  AffineConversion=off  FilteringAndDerivatives=provide  SimscapeFilterOrder=1  InputFilterTimeConstant=0.001  UdotUserProvided=0
  Thermal Reference : fl_lib/Thermal/Thermal Elements/Thermal Reference
  Conn1 : PMIOPort  Side=Left
  wires:
  Constant/1 -> Product/2
  Constant1/1 -> Product/1
  [SOL_EAST] -> Product/3
  Product/1 -> Add/1
  Constant3/1 -> Product1/1
  [SOL_SOUTH] -> Product1/3
  Constant2/1 -> Product1/2
  Add/1 -> Simulink-PS Converter/1
  Product1/1 -> Add/2
  connections:
  Controlled Heat Flow Rate Source/LConn1 -- Conn1/RConn1
  Simulink-PS Converter/RConn1 -- Controlled Heat Flow Rate Source/RConn1
  Thermal Reference/LConn1 -- Controlled Heat Flow Rate Source/RConn2

== system Task_No6_Thermal/sub_House/Kitchen/SOLAR__WINDOW ==
  Constant : Constant  Value=P_AREA_WIN_KIT
  Constant1 : Constant  Value=P_EM_GLASS
  Controlled Heat Flow Rate Source : fl_lib/Thermal/Thermal Sources/Controlled Heat Flow Rate Source
  Product : Product  Inputs=3
  Simulink-PS Converter : nesl_utility/Simulink-PS Converter  PhysicalDomain=network_engine_domain  SubClassName=ps_input  LeftPortType=input  RightPortType=output  PseudoPeriodic=off  Frequencies=[]  NoiseDistribution=none  NoiseParameters=[]  Unit=1  AffineConversion=off  FilteringAndDerivatives=provide  SimscapeFilterOrder=1  InputFilterTimeConstant=0.001  UdotUserProvided=0
  Thermal Reference : fl_lib/Thermal/Thermal Elements/Thermal Reference
  Conn1 : PMIOPort  Side=Left
  wires:
  Product/1 -> Simulink-PS Converter/1
  [SOL_SOUTH] -> Product/3
  Constant1/1 -> Product/1
  Constant/1 -> Product/2
  connections:
  Thermal Reference/LConn1 -- Controlled Heat Flow Rate Source/RConn2
  Simulink-PS Converter/RConn1 -- Controlled Heat Flow Rate Source/RConn1
  Controlled Heat Flow Rate Source/LConn1 -- Conn1/RConn1

== system Task_No6_Thermal/sub_House/Kitchen/TEMP_01 ==
  Constant2 : Constant  Value=Conv_C_to_K
  PS-Simulink Converter : nesl_utility/PS-Simulink Converter  PhysicalDomain=network_engine_domain  SubClassName=ps_output  LeftPortType=input  RightPortType=output  PseudoPeriodic=off  Frequencies=[]  VectorFormat=inherit  Unit=inherit  AffineConversion=off
  Sum : Sum  Inputs=|+-
  Temperature Sensor : fl_lib/Thermal/Thermal Sensors/Temperature Sensor  temperature_measure=foundation.enum.MeasurementReference.difference
  Thermal Reference2 : fl_lib/Thermal/Thermal Elements/Thermal Reference
  PS : PMIOPort  Side=Left
  Sim : Outport
  wires:
  Sum/1 -> Sim/1
  PS-Simulink Converter/1 -> Sum/1
  Constant2/1 -> Sum/2
  connections:
  Thermal Reference2/LConn1 -- Temperature Sensor/RConn1
  PS-Simulink Converter/LConn1 -- Temperature Sensor/RConn2
  PS/RConn1 -- Temperature Sensor/LConn1

== system Task_No6_Thermal/sub_House/Kitchen/Wall (KIT<->Outside) ==
  InAir-Wall : fl_lib/Thermal/Thermal Elements/Thermal Resistance  resistance=1/(U_WALL*P_AREA_OUTER_WALL_KIT)/2 K/W  T_specify=off  T_priority=None  T=0 K  T_nominal_specify=off  T_nominal_unit=K  T_nominal_value=1  Q_specify=off  Q_priority=None  Q=0 W  Q_nominal_specify=off  Q_nominal_unit=W  Q_nominal_value=1
  Thermal Mass of wall : fl_lib/Thermal/Thermal Elements/Thermal Mass  mass_type=foundation.enum.constant_variable.constant  mass=P_AREA_OUTER_WALL_KIT*(P_THICK_BRICK*P_DENSITY_BRICK+P_THICK_PUR*P_DENSITY_PUR) kg  sp_heat=P_CP_WALL J/(K*kg)  mass_min=1e-6 kg  num_ports=foundation.enum.numPorts2.one  m_specify=off  m_priority=High  m=1 kg  m_nominal_specify=off  m_nominal_unit=kg  m_nominal_value=1  T_specify=on  T_priority=High  T=T_INIT_BDR degC  T_nominal_specify=off  T_nominal_unit=K  T_nominal_value=1  Q_specify=off  Q_priority=None  Q=0 W  Q_nominal_specify=off  Q_nominal_unit=W  Q_nominal_value=1
  Wall-OutAir : fl_lib/Thermal/Thermal Elements/Thermal Resistance  resistance=1/(U_WALL*P_AREA_OUTER_WALL_KIT)/2 K/W  T_specify=off  T_priority=None  T=0 K  T_nominal_specify=off  T_nominal_unit=K  T_nominal_value=1  Q_specify=off  Q_priority=None  Q=0 W  Q_nominal_specify=off  Q_nominal_unit=W  Q_nominal_value=1
  Conn1 : PMIOPort  Side=Left
  Conn3 : PMIOPort  Port=2  Side=Right
  Conn2 : PMIOPort  Port=3  Side=Right
  connections:
  Conn1/RConn1 -- InAir-Wall/LConn1
  InAir-Wall/RConn1 -- Conn3/RConn1 -- Thermal Mass of wall/LConn1 -- Wall-OutAir/LConn1
  Wall-OutAir/RConn1 -- Conn2/RConn1

== system Task_No6_Thermal/sub_House/Kitchen/Window (KIT<->Outside) ==
  InAir-Window : fl_lib/Thermal/Thermal Elements/Thermal Resistance  resistance=1/(U_WINDOW*P_AREA_WIN_KIT)/2 K/W  T_specify=off  T_priority=None  T=0 K  T_nominal_specify=off  T_nominal_unit=K  T_nominal_value=1  Q_specify=off  Q_priority=None  Q=0 W  Q_nominal_specify=off  Q_nominal_unit=W  Q_nominal_value=1
  Thermal Mass of window : fl_lib/Thermal/Thermal Elements/Thermal Mass  mass_type=foundation.enum.constant_variable.constant  mass=P_M_WINDOW_SPEC*P_AREA_WIN_KIT kg  sp_heat=P_CP_GLASS J/(K*kg)  mass_min=1e-6 kg  num_ports=foundation.enum.numPorts2.one  m_specify=off  m_priority=High  m=1 kg  m_nominal_specify=off  m_nominal_unit=kg  m_nominal_value=1  T_specify=on  T_priority=High  T=T_INIT_BDR degC  T_nominal_specify=off  T_nominal_unit=K  T_nominal_value=1  Q_specify=off  Q_priority=None  Q=0 W  Q_nominal_specify=off  Q_nominal_unit=W  Q_nominal_value=1
  Window-OutAir : fl_lib/Thermal/Thermal Elements/Thermal Resistance  resistance=1/(U_WINDOW*P_AREA_WIN_KIT)/2 K/W  T_specify=off  T_priority=None  T=0 K  T_nominal_specify=off  T_nominal_unit=K  T_nominal_value=1  Q_specify=off  Q_priority=None  Q=0 W  Q_nominal_specify=off  Q_nominal_unit=W  Q_nominal_value=1
  Conn1 : PMIOPort  Side=Right
  Conn2 : PMIOPort  Port=2  Side=Left
  Conn3 : PMIOPort  Port=3  Side=Right
  connections:
  Thermal Mass of window/LConn1 -- Conn3/RConn1 -- Window-OutAir/LConn1 -- InAir-Window/RConn1
  Conn1/RConn1 -- Window-OutAir/RConn1
  Conn2/RConn1 -- InAir-Window/LConn1

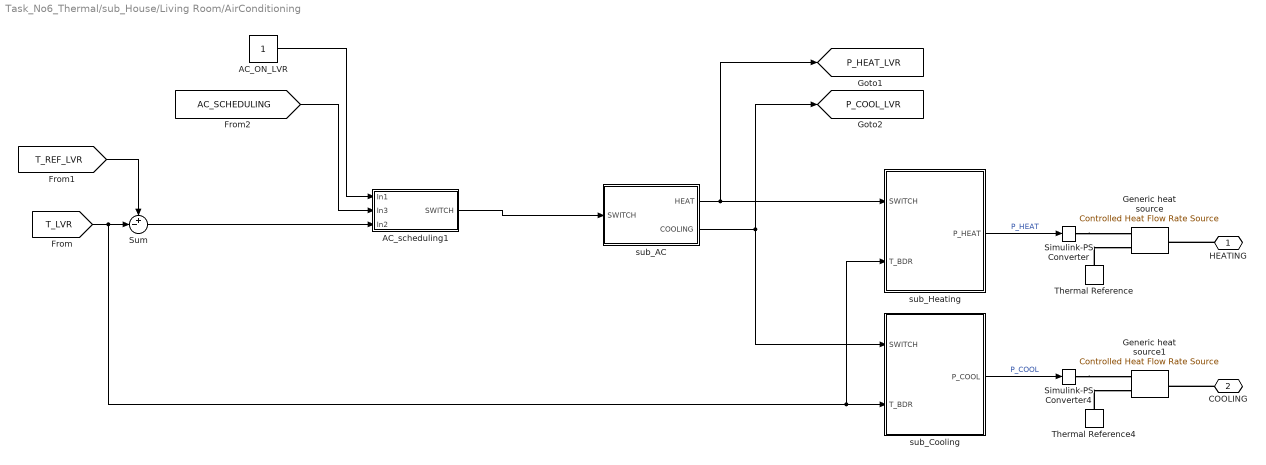
== system Task_No6_Thermal/sub_House/Living Room/AirConditioning ==
  AC_ON_LVR : Constant
  AC_scheduling1 : Subsystem
  Generic heat source : fl_lib/Thermal/Thermal Sources/Controlled Heat Flow Rate Source
  Generic heat source1 : fl_lib/Thermal/Thermal Sources/Controlled Heat Flow Rate Source
  Simulink-PS Converter : nesl_utility/Simulink-PS Converter  PhysicalDomain=network_engine_domain  SubClassName=ps_input  LeftPortType=input  RightPortType=output  PseudoPeriodic=off  Frequencies=[]  NoiseDistribution=none  NoiseParameters=[]  Unit=1  AffineConversion=off  FilteringAndDerivatives=provide  SimscapeFilterOrder=1  InputFilterTimeConstant=0.001  UdotUserProvided=0
  Simulink-PS Converter4 : nesl_utility/Simulink-PS Converter  PhysicalDomain=network_engine_domain  SubClassName=ps_input  LeftPortType=input  RightPortType=output  PseudoPeriodic=off  Frequencies=[]  NoiseDistribution=none  NoiseParameters=[]  Unit=1  AffineConversion=off  FilteringAndDerivatives=provide  SimscapeFilterOrder=1  InputFilterTimeConstant=0.001  UdotUserProvided=0
  Sum : Sum  Inputs=+-|
  Thermal Reference : fl_lib/Thermal/Thermal Elements/Thermal Reference
  Thermal Reference4 : fl_lib/Thermal/Thermal Elements/Thermal Reference
  sub_AC : Subsystem
  sub_Cooling : Subsystem
  sub_Heating : Subsystem
  HEATING : PMIOPort  Side=Right
  COOLING : PMIOPort  Port=2  Side=Right
  tag scope: P_COOL_LVR=global, P_HEAT_LVR=global
  wires:
  sub_AC/2(COOLING) -> [P_COOL_LVR], sub_Cooling/1(SWITCH)
  sub_AC/1(HEAT) -> [P_HEAT_LVR], sub_Heating/1(SWITCH)
  [T_LVR] -> sub_Heating/2(T_BDR), sub_Cooling/2(T_BDR), Sum/2
  sub_Heating/1(P_HEAT) -> Simulink-PS Converter/1  "P_HEAT"
  sub_Cooling/1(P_COOL) -> Simulink-PS Converter4/1  "P_COOL"
  [T_REF_LVR] -> Sum/1
  AC_scheduling1/1(SWITCH) -> sub_AC/1(SWITCH)
  AC_ON_LVR/1 -> AC_scheduling1/1(In1)
  [AC_SCHEDULING] -> AC_scheduling1/2(In3)
  Sum/1 -> AC_scheduling1/3(In2)
  connections:
  Thermal Reference4/LConn1 -- Generic heat source1/RConn2
  Thermal Reference/LConn1 -- Generic heat source/RConn2
  Simulink-PS Converter4/RConn1 -- Generic heat source1/RConn1
  Simulink-PS Converter/RConn1 -- Generic heat source/RConn1
  HEATING/RConn1 -- Generic heat source/LConn1
  COOLING/RConn1 -- Generic heat source1/LConn1

== system Task_No6_Thermal/sub_House/Living Room/Ceiling & Floor (LVR<->Above & Below) ==
  Ceiling-InAir : fl_lib/Thermal/Thermal Elements/Thermal Resistance  resistance=1/(U_CEIL*P_AREA_LVR) K/W  T_specify=off  T_priority=None  T=0 K  T_nominal_specify=off  T_nominal_unit=K  T_nominal_value=1  Q_specify=off  Q_priority=None  Q=0 W  Q_nominal_specify=off  Q_nominal_unit=W  Q_nominal_value=1
  Floor-InAir : fl_lib/Thermal/Thermal Elements/Thermal Resistance  resistance=1/(U_CEIL*P_AREA_LVR) K/W  T_specify=off  T_priority=None  T=0 K  T_nominal_specify=off  T_nominal_unit=K  T_nominal_value=1  Q_specify=off  Q_priority=None  Q=0 W  Q_nominal_specify=off  Q_nominal_unit=W  Q_nominal_value=1
  Conn1 : PMIOPort  Side=Left
  Conn2 : PMIOPort  Port=2  Side=Right
  connections:
  Conn1/RConn1 -- Ceiling-InAir/LConn1 -- Floor-InAir/LConn1
  Conn2/RConn1 -- Ceiling-InAir/RConn1 -- Floor-InAir/RConn1
